simulink model "switch_model"  (Simulink 5.0)
settings: Solver=FixedStepDiscrete  StartTime=0.0  StopTime=10.0  RelTol=1e-3
settings Model: Creator=sofronis  LastModifiedBy=sofronis  ExtModeAutoUpdateStatusClock=off  AlgebraicLoopMsg=error

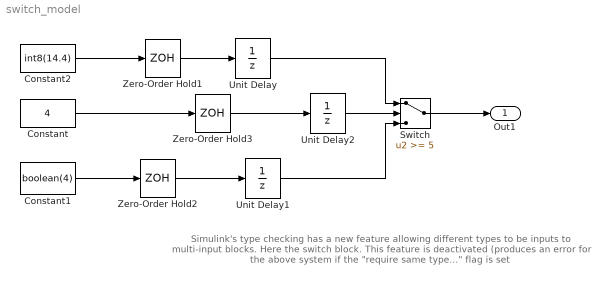
== system switch_model ==
  note: Simulink's type checking has a new feature allowing different
      | types to be inputs to multi-input blocks. Here the
      | switch block.
      |
      | This feature is deactivated (produces an error for
      | the above system if the "require same type..." flag
      | is set
  Constant : Constant  Value=4
  Constant1 : Constant  Value=boolean(4)
  Constant2 : Constant  Value=int8(14.4)
  Switch : Switch  Threshold=5  ShowAdditionalParam=on  SaturateOnIntegerOverflow=on
  Unit Delay : UnitDelay  SampleTime=-1
  Unit Delay1 : UnitDelay  SampleTime=-1
  Unit Delay2 : UnitDelay  SampleTime=-1
  Zero-Order Hold1 : ZeroOrderHold  SampleTime=2
  Zero-Order Hold2 : ZeroOrderHold
  Zero-Order Hold3 : ZeroOrderHold  SampleTime=9
  Out1 : Outport
  wires:
  Constant/1 -> Zero-Order Hold3/1
  Constant1/1 -> Zero-Order Hold2/1
  Switch/1 -> Out1/1
  Constant2/1 -> Zero-Order Hold1/1
  Zero-Order Hold1/1 -> Unit Delay/1
  Zero-Order Hold2/1 -> Unit Delay1/1
  Unit Delay/1 -> Switch/1
  Unit Delay1/1 -> Switch/3
  Zero-Order Hold3/1 -> Unit Delay2/1
  Unit Delay2/1 -> Switch/2
